simulink model "sm_ssci_hydraulic_lift_trsn"  (R2021b)
settings: Solver=VariableStepAuto  StartTime=0.0  StopTime=30  RelTol=1e-3  AbsTol=1e-3  EnableMultiTasking=on
PostLoadFcn:
  | warning off sm:compiler:state:UnsatisfiedDesiredTarget
  | warning off Simulink:Engine:UsingDefaultMaxStepSize
  | warning('off','sm:sli:setup:compile:SteadyStateStartNotSupported')
model workspace (MATLAB code in the model file):
  | % Units of cm
  | cyl_len = 11;
  | cyl_rOut = 1.1;
  | cyl_rInn = 1;
  | cap_len = 1;
  | 
  | pst_len = 1;
  | pst_rOut = cyl_rInn;
  | 
  | rod_len = 14;
  | rod_rOut = 0.5;
  | 
  | leg_length = 15;
  | platform_length = 25;
undefined symbols (not defined in the file or in its folder): X, Y, Z
libraries: sm_lib x21, fl_lib x12, nesl_utility x3, Multibody_Multiphysics_Lib x1, simulink x1
(part 2 of 2)

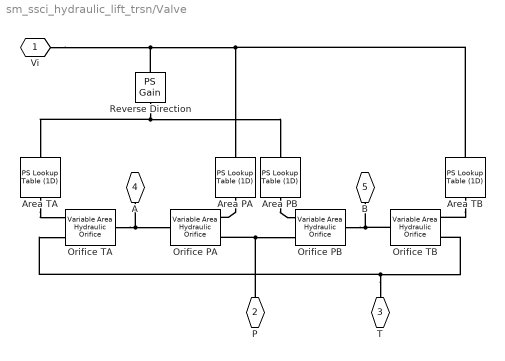
== system sm_ssci_hydraulic_lift_trsn/Valve ==
  Area PA : fl_lib/Physical Signals/Lookup Tables/PS Lookup Table (1D)  x=[-x_max -x_lap 0 x_lap x_max 2*x_max]  f=[0 0 A_leak 2*A_leak A_max A_max]*1e-6  interp_method=1  extrap_method=1
      settings: SourceProductBaseCode=SS
  Area PB : fl_lib/Physical Signals/Lookup Tables/PS Lookup Table (1D)  x=[-x_max -x_lap 0 x_lap x_max 2*x_max]  f=[0 0 A_leak 2*A_leak A_max A_max]*1e-6  interp_method=1  extrap_method=1
      settings: SourceProductBaseCode=SS
  Area TA : fl_lib/Physical Signals/Lookup Tables/PS Lookup Table (1D)  x=[-x_max -x_lap 0 x_lap x_max 2*x_max]  f=[0 0 A_leak 2*A_leak A_max A_max]*1e-6  interp_method=1  extrap_method=1
      settings: SourceProductBaseCode=SS
  Area TB : fl_lib/Physical Signals/Lookup Tables/PS Lookup Table (1D)  x=[-x_max -x_lap 0 x_lap x_max 2*x_max]  f=[0 0 A_leak 2*A_leak A_max A_max]*1e-6  interp_method=1  extrap_method=1
      settings: SourceProductBaseCode=SS
  Orifice PA : fl_lib/Hydraulic/Hydraulic Elements/Variable Area Hydraulic Orifice  C_d=K_V  min_area=1e-12 m^2  lam_spec=2  B_lam=0.999  Re_cr=12  q_specify=off  q_priority=High  q=1 m^3/s  q_nominal_specify=off  q_nominal_unit=m^3/s  q_nominal_value=1  p_specify=off  p_priority=High  p=0 Pa  p_nominal_specify=off  p_nominal_unit=Pa  p_nominal_value=1
      settings: SourceProductBaseCode=SS  InternalSimscapePortConfiguration="{\"Bottom\":[],\"Left\":[{\"id\":\"AR\",\"label\":\"AR\",\"type\":\"input\"},{\"id\":\"A\",\"label\":\"A\",\"type\":\"foundation.hydraulic.hydraulic\"}],\"Right\":[{\"id\":\"B\",\"label\":\"B\",\"type\":\"foundation.hydraulic.hydraulic\"}],\"Top\":[]}"
  Orifice PB : fl_lib/Hydraulic/Hydraulic Elements/Variable Area Hydraulic Orifice  C_d=K_V  min_area=1e-12 m^2  lam_spec=2  B_lam=0.999  Re_cr=12  q_specify=off  q_priority=High  q=1 m^3/s  q_nominal_specify=off  q_nominal_unit=m^3/s  q_nominal_value=1  p_specify=off  p_priority=High  p=0 Pa  p_nominal_specify=off  p_nominal_unit=Pa  p_nominal_value=1
      settings: SourceProductBaseCode=SS  InternalSimscapePortConfiguration="{\"Bottom\":[],\"Left\":[{\"id\":\"AR\",\"label\":\"AR\",\"type\":\"input\"},{\"id\":\"A\",\"label\":\"A\",\"type\":\"foundation.hydraulic.hydraulic\"}],\"Right\":[{\"id\":\"B\",\"label\":\"B\",\"type\":\"foundation.hydraulic.hydraulic\"}],\"Top\":[]}"
  Orifice TA : fl_lib/Hydraulic/Hydraulic Elements/Variable Area Hydraulic Orifice  C_d=K_V  min_area=1e-12 m^2  lam_spec=2  B_lam=0.999  Re_cr=12  q_specify=off  q_priority=High  q=1 m^3/s  q_nominal_specify=off  q_nominal_unit=m^3/s  q_nominal_value=1  p_specify=off  p_priority=High  p=0 Pa  p_nominal_specify=off  p_nominal_unit=Pa  p_nominal_value=1
      settings: SourceProductBaseCode=SS  InternalSimscapePortConfiguration="{\"Bottom\":[],\"Left\":[{\"id\":\"AR\",\"label\":\"AR\",\"type\":\"input\"},{\"id\":\"A\",\"label\":\"A\",\"type\":\"foundation.hydraulic.hydraulic\"}],\"Right\":[{\"id\":\"B\",\"label\":\"B\",\"type\":\"foundation.hydraulic.hydraulic\"}],\"Top\":[]}"
  Orifice TB : fl_lib/Hydraulic/Hydraulic Elements/Variable Area Hydraulic Orifice  C_d=K_V  min_area=1e-12 m^2  lam_spec=2  B_lam=0.999  Re_cr=12  q_specify=off  q_priority=High  q=1 m^3/s  q_nominal_specify=off  q_nominal_unit=m^3/s  q_nominal_value=1  p_specify=off  p_priority=High  p=0 Pa  p_nominal_specify=off  p_nominal_unit=Pa  p_nominal_value=1
      settings: SourceProductBaseCode=SS  InternalSimscapePortConfiguration="{\"Bottom\":[],\"Left\":[{\"id\":\"AR\",\"label\":\"AR\",\"type\":\"input\"},{\"id\":\"A\",\"label\":\"A\",\"type\":\"foundation.hydraulic.hydraulic\"}],\"Right\":[{\"id\":\"B\",\"label\":\"B\",\"type\":\"foundation.hydraulic.hydraulic\"}],\"Top\":[]}"
  Reverse Direction : fl_lib/Physical Signals/Functions/PS Gain  gain=-1
  Vi : PMIOPort  Tag=PMCPort  Side=Left
  P : PMIOPort  Tag=PMCPort  Port=2  Side=Left
  T : PMIOPort  Tag=PMCPort  Port=3  Side=Left
  A : PMIOPort  Tag=PMCPort  Port=4  Side=Right
  B : PMIOPort  Tag=PMCPort  Port=5  Side=Right
  connections:
  B/RConn1 -- Orifice PB/RConn1 -- Orifice TB/RConn1
  T/RConn1 -- Orifice TA/LConn2 -- Orifice TB/LConn2
  A/RConn1 -- Orifice PA/RConn1 -- Orifice TA/RConn1
  P/RConn1 -- Orifice PA/LConn2 -- Orifice PB/LConn2
  Reverse Direction/RConn1 -- Area PB/LConn1 -- Area TA/LConn1
  Area TB/RConn1 -- Orifice TB/LConn1
  Area PA/RConn1 -- Orifice PA/LConn1
  Vi/RConn1 -- Reverse Direction/LConn1 -- Area TB/LConn1 -- Area PA/LConn1
  Area TA/RConn1 -- Orifice TA/LConn1
  Area PB/RConn1 -- Orifice PB/LConn1

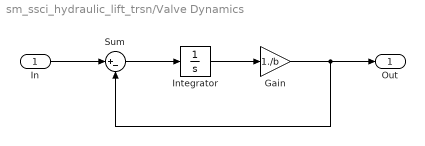
== system sm_ssci_hydraulic_lift_trsn/Valve Dynamics ==
  In : Inport
  Gain : Gain  Gain=1./b
  Integrator : Integrator  InitialCondition=x_initial.*b
  Sum : Sum  Inputs=|+-  InputSameDT=on  SaturateOnIntegerOverflow=on  OutDataTypeStr=Inherit: Same as first input
  Out : Outport  VectorParamsAs1DForOutWhenUnconnected=off
  wires:
  Sum/1 -> Integrator/1
  In/1 -> Sum/1
  Integrator/1 -> Gain/1
  Gain/1 -> Sum/2, Out/1
